simulink model "untitled"  (R2022b)
settings: Solver=VariableStepAuto  StartTime=0.0  StopTime=10.0  RelTol=1e-3

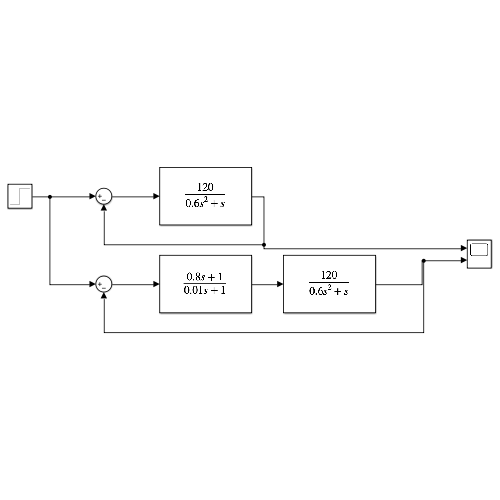
[thumbnail: Simulink's stored preview of the top-level diagram]
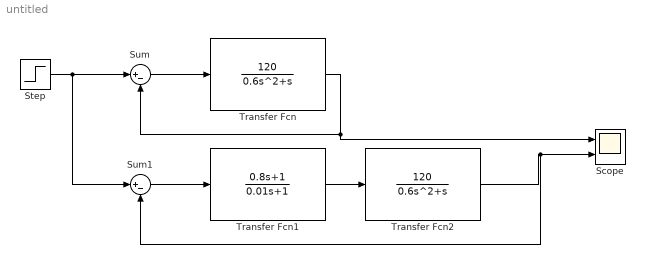
== system untitled ==
  Scope : Scope  NumInputPorts=2
  Step : Step  SampleTime=0
  Sum : Sum  Inputs=|+-
  Sum1 : Sum  Inputs=|+-
  Transfer Fcn : TransferFcn  Numerator=[120]  Denominator=[0.6 1 0]
  Transfer Fcn1 : TransferFcn  Numerator=[0.8 1]  Denominator=[0.01 1]
  Transfer Fcn2 : TransferFcn  Numerator=[120]  Denominator=[0.6 1 0]
  wires:
  Transfer Fcn/1 -> Sum/2, Scope/1
  Sum/1 -> Transfer Fcn/1
  Sum1/1 -> Transfer Fcn1/1
  Step/1 -> Sum1/1, Sum/1
  Transfer Fcn1/1 -> Transfer Fcn2/1
  Transfer Fcn2/1 -> Sum1/2, Scope/2
